simulink model "Opg_8_2_simulink"  (R2020a)
settings: Solver=VariableStepAuto  StartTime=0.0  StopTime=5  RelTol=1e-3
PreLoadFcn:
  | Opg_8_2_matlab
values from neighbouring files (symbols this model uses):
  Kp = 5    [Opg_8_2_AfterSolutionExample.m]    (also in handinTemplate.m = 1)
  N = 30    [Opg_8_2_AfterSolutionExample.m]
  T = 1/100    (= 0.01)    [Opg_8_2_AfterSolutionExample.m]    (also in Opg_9_2.m = 0.05; Opg_9_3.m = inv(invT))
  Td = 1    [Opg_8_2_AfterSolutionExample.m]    (also in handinTemplate.m = 0.025)
undefined symbols (not defined in the file or in its folder): Gdden, Gden, Gdnum, Gnum, Kden, Knum, T2, T3
settings Model: Creator=Emil  LastModifiedBy=Emil

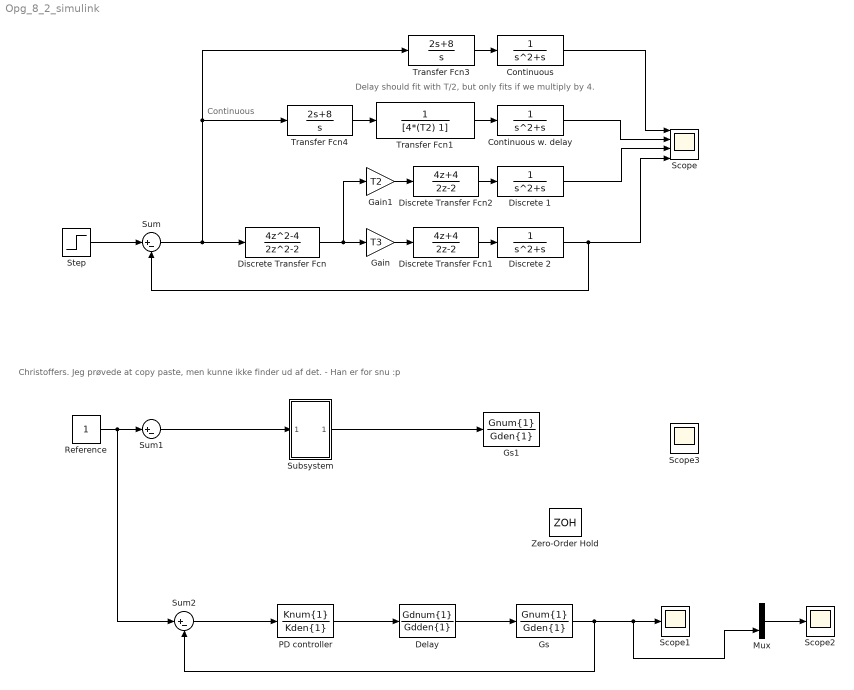
== system Opg_8_2_simulink ==
  note: Christoffers. Jeg prøvede at copy paste, men kunne ikke finder ud af det. - Han er for snu :p
  note: Delay should fit with T/2, but only fits if we multiply by 4.
  note: Continuous
  Continuous : TransferFcn  Denominator=[1 1 0]
  Continuous w. delay : TransferFcn  Denominator=[1 1 0]
  Delay : TransferFcn  Numerator=Gdnum{1}  Denominator=Gdden{1}
  Discrete Transfer Fcn : DiscreteTransferFcn  Numerator=[4 0 -4]  Denominator=[2 0 -2]
  Discrete Transfer Fcn1 : DiscreteTransferFcn  Numerator=[4 4]  Denominator=[2 -2]
  Discrete Transfer Fcn2 : DiscreteTransferFcn  Numerator=[4 4]  Denominator=[2 -2]
  Discrete 1 : TransferFcn  Denominator=[1 1 0]
  Discrete 2 : TransferFcn  Denominator=[1 1 0]
  Gain : Gain  Gain=T3
  Gain1 : Gain  Gain=T2
  Gs : TransferFcn  Numerator=Gnum{1}  Denominator=Gden{1}
  Gs1 : TransferFcn  Numerator=Gnum{1}  Denominator=Gden{1}
  Mux : Mux  Inputs=2
  PD controller : TransferFcn  Numerator=Knum{1}  Denominator=Kden{1}
  Reference : Constant
  Scope : Scope  NumInputPorts=4
  Scope1 : Scope
  Scope2 : Scope
  Scope3 : Scope
  Step : Step  SampleTime=0
  Subsystem : Subsystem
  Sum : Sum  Inputs=|+-
  Sum1 : Sum  Inputs=|+-
  Sum2 : Sum  Inputs=|+-
  Transfer Fcn1 : TransferFcn  Denominator=[4*(T2) 1]
  Transfer Fcn3 : TransferFcn  Numerator=[2 8]  Denominator=[1 0]
  Transfer Fcn4 : TransferFcn  Numerator=[2 8]  Denominator=[1 0]
  Zero-Order Hold : ZeroOrderHold  SampleTime=T
  wires:
  Step/1 -> Sum/1
  Discrete 2/1 -> Scope/4, Sum/2
  Discrete Transfer Fcn1/1 -> Discrete 2/1
  Gain/1 -> Discrete Transfer Fcn1/1
  Gain1/1 -> Discrete Transfer Fcn2/1
  Discrete Transfer Fcn2/1 -> Discrete 1/1
  Discrete Transfer Fcn/1 -> Gain1/1, Gain/1
  Sum/1 -> Transfer Fcn3/1, Transfer Fcn4/1, Discrete Transfer Fcn/1
  Transfer Fcn1/1 -> Continuous w. delay/1
  Transfer Fcn4/1 -> Transfer Fcn1/1
  Transfer Fcn3/1 -> Continuous/1
  Discrete 1/1 -> Scope/3
  Continuous w. delay/1 -> Scope/2
  Continuous/1 -> Scope/1
  Reference/1 -> Sum2/1, Sum1/1
  PD controller/1 -> Delay/1
  Delay/1 -> Gs/1
  Sum2/1 -> PD controller/1
  Gs/1 -> Sum2/2, Mux/2, Scope1/1
  Mux/1 -> Scope2/1
  Sum1/1 -> Subsystem/1(In1)
  Subsystem/1(Out1) -> Gs1/1

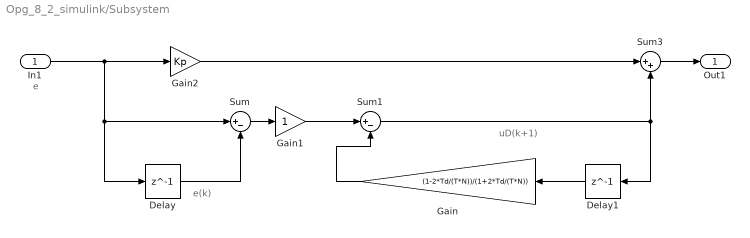
== system Opg_8_2_simulink/Subsystem ==
  note: uD(k+1)
  note: e(k)
  note: e
  In1 : Inport
  Delay : Delay  DelayLength=1
  Delay1 : Delay  DelayLength=1
  Gain : Gain  Gain=(1-2*Td/(T*N))/(1+2*Td/(T*N))
  Gain1 : Gain
  Gain2 : Gain  Gain=Kp
  Sum : Sum  Inputs=|+-
  Sum1 : Sum  Inputs=|+-
  Sum3 : Sum  Inputs=|++
  Out1 : Outport
  wires:
  Gain2/1 -> Sum3/1
  Sum3/1 -> Out1/1
  In1/1 -> Delay/1, Sum/1, Gain2/1
  Sum1/1 -> Sum3/2, Delay1/1
  Delay/1 -> Sum/2
  Delay1/1 -> Gain/1
  Sum/1 -> Gain1/1
  Gain1/1 -> Sum1/1
  Gain/1 -> Sum1/2
